simulink model "PLANTA_CODESYS"  (R2024b)
settings: Solver=FixedStepAuto  StartTime=0.0  StopTime=inf  FixedStep=0.001  MaxStep=0.0005  RelTol=1e-4
undefined symbols (not defined in the file): A_hm, A_tm, at_breakpoints, b_ha, B_hm, b_ta, B_tm, bcx, bcy, bhd, bhEb, bhm, bt, btd, btm, btw, bwu, C_hm, C_tm, D_hm, D_tm, DiscIntNeverNeededParam, dl_h_ini, dx_l_ini, dx_t_ini, dx_td_ini, dxt_max, dy_l_ini, g, Hc, ih, it, J_eqt, Jhd_hEb, Jhm_hb, Jtd, Jtm_tb, K_hsa, K_hsia, K_tsa, K_tsia, Kcy, Kd_table, ke_int, Ke_tita, ke_tita, ke_w, Ke_w, kp_pos, Kp_table, kp_w, kpos, Ktw, kwu, l_breakpoints, l_h_ini, Lh0, ml_breakpoints, Ms, Mt ... (+16)
libraries: simulink x11, spsEdgeDetectorLib x5, simulink_extras x2, opcualib x2, dspsigops x2, dspstat3 x1, vrlib x1, sldrtlib x1
(part 2 of 2)

== system PLANTA_CODESYS/PLANTA/Altura perfil obstaculos (A partir de posicion x_l) ==
  x_l : Inport
  Ajuste referencia : Constant  Value=30
  Calculo : MATLAB Function  TreatAsAtomicUnit=on
  Data Store Read : DataStoreRead  DataStoreName=y0_global  IndexOptions=Index vector (dialog)  Indices=1  OutputSizes=1
  Data Type Conversion : DataTypeConversion  OutDataTypeStr=int32  RndMeth=Ceiling  SaturateOnIntegerOverflow=off
  Gain1 : Gain  Gain=1/Wc
  Scope : Scope
  Scope1 : Scope
  Sum : Sum  Inputs=|++
  yc0_xl : Outport
  wires:
  Calculo/1(yc0_xt) -> Scope1/1, yc0_xl/1
  Data Store Read/1 -> Calculo/1(y0_array)
  Data Type Conversion/1 -> Scope/1, Calculo/2(index)
  Gain1/1 -> Data Type Conversion/1
  Ajuste referencia/1 -> Sum/2
  Sum/1 -> Gain1/1
  x_l/1 -> Sum/1

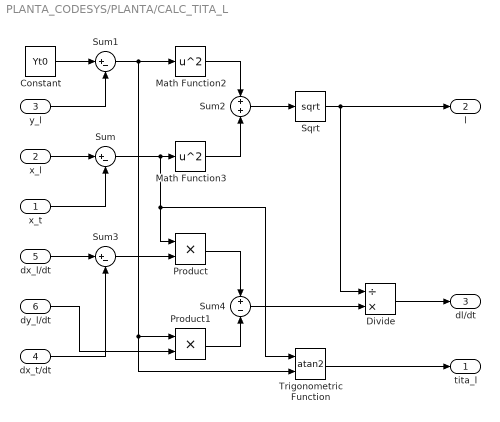
== system PLANTA_CODESYS/PLANTA/CALC_TITA_L ==
  x_t : Inport
  x_l : Inport  Port=2
  y_l : Inport  Port=3
  dx_t/dt : Inport  Port=4
  dx_l/dt : Inport  Port=5
  dy_l/dt : Inport  Port=6
  Constant : Constant  Value=Yt0
  Divide : Product  Inputs=/*
  Math Function2 : Math  Operator=square
  Math Function3 : Math  Operator=square
  Product : Product
  Product1 : Product
  Sqrt : Sqrt
  Sum : Sum  Inputs=|+-
  Sum1 : Sum  Inputs=|+-
  Sum2 : Sum  Inputs=+|+
  Sum3 : Sum  Inputs=|+-
  Sum4 : Sum  Inputs=+|-
  Trigonometric Function : Trigonometry  Operator=atan2
  tita_l : Outport
  l : Outport  Port=2
  dl/dt : Outport  Port=3
  wires:
  Product/1 -> Sum4/1
  Product1/1 -> Sum4/2
  x_l/1 -> Sum/1
  dx_t/dt/1 -> Sum3/2
  y_l/1 -> Sum1/2
  Sum/1 -> Product/1, Trigonometric Function/1, Math Function3/1
  Sqrt/1 -> l/1, Divide/1
  Sum2/1 -> Sqrt/1
  Sum4/1 -> Divide/2
  Sum1/1 -> Product1/1, Trigonometric Function/2, Math Function2/1
  Math Function2/1 -> Sum2/1
  dx_l/dt/1 -> Sum3/1
  x_t/1 -> Sum/2
  Constant/1 -> Sum1/1
  Sum3/1 -> Product/2
  dy_l/dt/1 -> Product1/2
  Math Function3/1 -> Sum2/2
  Trigonometric Function/1 -> tita_l/1
  Divide/1 -> dl/dt/1

== system PLANTA_CODESYS/PLANTA/FIN_CARRERA_IZAJE ==
  l_h : Inport
  Constant : Constant  Value=Yt0
  Constant1 : Constant  Value=-19.5
  Constant2 : Constant  Value=-20
  Constant3 : Constant  Value=49.5
  Constant4 : Constant  Value=50
  Relational Operator : RelationalOperator  Operator=<=  OutDataTypeStr=boolean  RndMeth=Simplest  InputSameDT=off
  Relational Operator1 : RelationalOperator  Operator=<=  OutDataTypeStr=boolean  RndMeth=Simplest  InputSameDT=off
  Relational Operator2 : RelationalOperator  OutDataTypeStr=boolean  RndMeth=Simplest  InputSameDT=off
  Relational Operator3 : RelationalOperator  OutDataTypeStr=boolean  RndMeth=Simplest  InputSameDT=off
  Sum : Sum  Inputs=|-+
  FC_INF : Outport
  FCE_INF : Outport  Port=2
  FC_SUP : Outport  Port=3
  FCE_SUP : Outport  Port=4
  wires:
  Sum/1 -> Relational Operator3/1, Relational Operator2/1, Relational Operator/1, Relational Operator1/1  "y_h"
  Relational Operator3/1 -> FCE_SUP/1
  Constant4/1 -> Relational Operator3/2
  Relational Operator2/1 -> FC_SUP/1
  Constant3/1 -> Relational Operator2/2
  Constant1/1 -> Relational Operator/2
  Constant2/1 -> Relational Operator1/2
  Relational Operator/1 -> FC_INF/1
  Constant/1 -> Sum/2
  Relational Operator1/1 -> FCE_INF/1
  l_h/1 -> Sum/1

== system PLANTA_CODESYS/PLANTA/Fin de carrera Carro ==
  x_t : Inport
  Constant : Constant  Value=-29.5
  Constant1 : Constant  Value=-30
  Constant2 : Constant  Value=49.5
  Constant3 : Constant  Value=50
  Relational Operator : RelationalOperator  Operator=<=  OutDataTypeStr=boolean  RndMeth=Simplest  InputSameDT=off
  Relational Operator1 : RelationalOperator  Operator=<=  OutDataTypeStr=boolean  RndMeth=Simplest  InputSameDT=off
  Relational Operator2 : RelationalOperator  OutDataTypeStr=boolean  RndMeth=Simplest  InputSameDT=off
  Relational Operator3 : RelationalOperator  OutDataTypeStr=boolean  RndMeth=Simplest  InputSameDT=off
  FC_IZQ : Outport
  FCE_IZQ : Outport  Port=2
  FC_DER : Outport  Port=3
  FCE_DER : Outport  Port=4
  wires:
  Relational Operator/1 -> FC_IZQ/1
  Constant1/1 -> Relational Operator1/2
  x_t/1 -> Relational Operator3/1, Relational Operator2/1, Relational Operator/1, Relational Operator1/1
  Relational Operator1/1 -> FCE_IZQ/1
  Constant2/1 -> Relational Operator2/2
  Relational Operator2/1 -> FC_DER/1
  Relational Operator3/1 -> FCE_DER/1
  Constant3/1 -> Relational Operator3/2
  Constant/1 -> Relational Operator/2

== system PLANTA_CODESYS/PLANTA/Fuerzas de tension de cable en Carro ==
  x_td : Inport
  dx_td : Inport  Port=2
  x_t : Inport  Port=3
  dx_t : Inport  Port=4
  Add : Sum  Inputs=+-
  Add1 : Sum  Inputs=+-
  Add2 : Sum
  Gain : Gain  Gain=Ktw
  Gain1 : Gain  Gain=btw
  F_tw : Outport
  wires:
  Add1/1 -> Gain1/1
  Add/1 -> Gain/1
  Gain1/1 -> Add2/2
  x_td/1 -> Add/1
  dx_t/1 -> Add1/2
  dx_td/1 -> Add1/1
  Gain/1 -> Add2/1
  Add2/1 -> F_tw/1
  x_t/1 -> Add/2

== system PLANTA_CODESYS/PLANTA/Masa de contenedor (A partir de posicion x_l) ==
  TLK : Inport
  x_l : Inport  Port=2
  masas_array : Inport  Port=3
  Ajuste referencia : Constant  Value=30
  Calculo : MATLAB Function  TreatAsAtomicUnit=on
  Data Type Conversion : DataTypeConversion  OutDataTypeStr=int32  RndMeth=Ceiling  SaturateOnIntegerOverflow=off
  Edge Detector : spsEdgeDetectorLib/Edge Detector  model=Falling  ic=0  Ts=-1
  Edge Detector1 : spsEdgeDetectorLib/Edge Detector  model=Rising  ic=0  Ts=-1
  Gain1 : Gain  Gain=1/Wc
  Product : Product
  S-R Flip-Flop : simulink_extras/Flip Flops/S-R Flip-Flop  initial_condition=0
  Sample and Hold : dspsigops/Sample and Hold  trig=Rising edge  initCond=0  latchinput=off
  Sum : Sum  Inputs=|++
  Unit Delay : UnitDelay  SampleTime=-1  HasFrameUpgradeWarning=on
  Mc_X : Outport
  wires:
  Data Type Conversion/1 -> Calculo/2(index)
  Gain1/1 -> Data Type Conversion/1
  Ajuste referencia/1 -> Sum/2
  Sum/1 -> Gain1/1
  x_l/1 -> Sum/1
  TLK/1 -> Unit Delay/1
  Edge Detector/1 -> S-R Flip-Flop/2
  Edge Detector1/1 -> S-R Flip-Flop/1
  S-R Flip-Flop/1 -> Sample and Hold/Trigger, Product/2
  Product/1 -> Mc_X/1
  Unit Delay/1 -> Edge Detector1/1, Edge Detector/1
  Calculo/1(Mc_X) -> Sample and Hold/1
  Sample and Hold/1 -> Product/1
  masas_array/1 -> Calculo/1(masas_array)

== system PLANTA_CODESYS/PLANTA/PERFIL_OBSTACULOS ==
  note: LIDAR
  x_t : Inport
  Ajuste distancia LIDAR : dspsigops/Variable Fractional Delay  mode=OBSOLETE  modeActive=Linear  L=4  FarrowL=4  R=10  alpha=1  dmax=100  InputProcessing=Columns as channels (frame based)  ic=0  noDFT=off  fallbackFIR=Clip to the minimum value necessary for centered kernel  fallbackFarrow=Clip to the minimum value necessary for centered kernel  roundingMode=Zero  overflowMode=off
  Ajuste referencia : Constant  Value=30
  Constant : Constant  Value=Yt0
  Data Type Conversion : DataTypeConversion  OutDataTypeStr=int32  RndMeth=Ceiling  SaturateOnIntegerOverflow=off
  Delay : Delay  DelayLength=1  InputProcessing=Columns as channels (frame based)  SampleTime=0.001
  Delay espacial : Constant  Value=3/Wc
  Gain : Gain  Gain=1/Wc
  Perfil obstaculos (ENTORNO) : FromWorkspace  VariableName=y0
  Posicion LIDAR : Constant  Value=3
  Sum : Sum  Inputs=|++
  Sum1 : Sum  Inputs=|++
  Sum2 : Sum  Inputs=+-|
  sensor : MATLAB Function  TreatAsAtomicUnit=on
  yc0_xt : Outport
  wires:
  Delay/1 -> Sum1/1
  Sum/1 -> Gain/1
  Constant/1 -> Sum2/1
  Sum2/1 -> yc0_xt/1
  Sum1/1 -> Sum/1
  Delay espacial/1 -> Ajuste distancia LIDAR/2
  Ajuste distancia LIDAR/1 -> Sum2/2
  Data Type Conversion/1 -> sensor/2(index)
  Perfil obstaculos (ENTORNO)/1 -> sensor/1(y0_array)
  sensor/1(distancia) -> Ajuste distancia LIDAR/1
  Posicion LIDAR/1 -> Sum1/2
  Gain/1 -> Data Type Conversion/1
  x_t/1 -> Delay/1
  Ajuste referencia/1 -> Sum/2

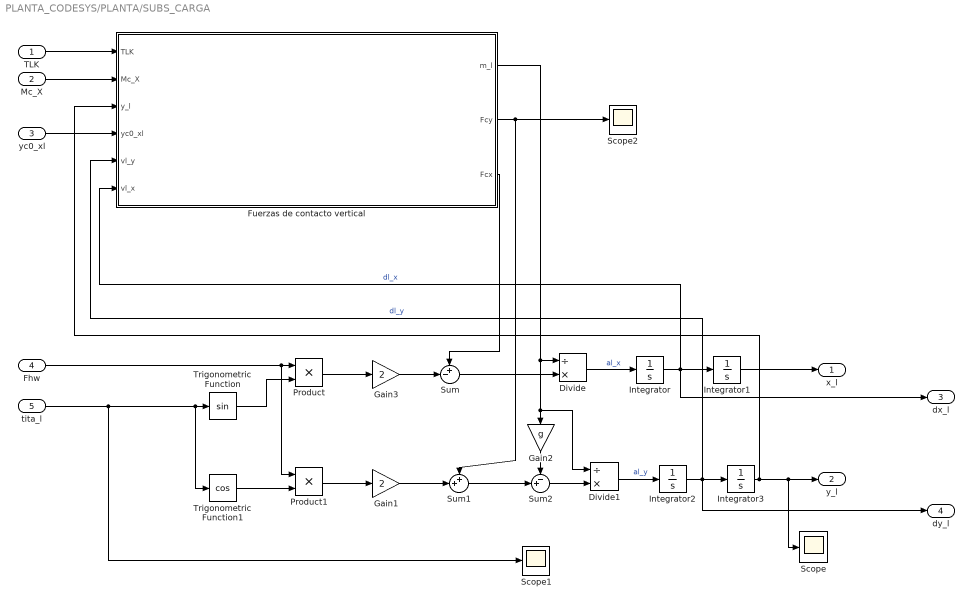
== system PLANTA_CODESYS/PLANTA/SUBS_CARGA ==
  TLK : Inport
  Mc_X : Inport  Port=2
  yc0_xl : Inport  Port=3
  Fhw : Inport  Port=4
  tita_l : Inport  Port=5
  Divide : Product  Inputs=/*
  Divide1 : Product  Inputs=/*
  Fuerzas de contacto vertical : Subsystem
  Gain1 : Gain  Gain=2
  Gain2 : Gain  Gain=g
  Gain3 : Gain  Gain=2
  Integrator : Integrator  InitialCondition=dx_l_ini
  Integrator1 : Integrator  InitialCondition=x_l_ini
  Integrator2 : Integrator  InitialCondition=dy_l_ini
  Integrator3 : Integrator  InitialCondition=y_l_ini
  Product : Product
  Product1 : Product
  Scope : Scope
  Scope1 : Scope
  Scope2 : Scope
  Sum : Sum  Inputs=+-|
  Sum1 : Sum  Inputs=++|
  Sum2 : Sum  Inputs=-+|
  Trigonometric Function : Trigonometry
  Trigonometric Function1 : Trigonometry  Operator=cos
  x_l : Outport
  y_l : Outport  Port=2
  dx_l : Outport  Port=3
  dy_l : Outport  Port=4
  wires:
  Divide1/1 -> Integrator2/1  "al_y"
  Sum2/1 -> Divide1/2
  Integrator2/1 -> dy_l/1, Integrator3/1, Fuerzas de contacto vertical/5(vl_y)  "dl_y"
  Fhw/1 -> Product1/1, Product/1
  Integrator3/1 -> Scope/1, y_l/1, Fuerzas de contacto vertical/3(y_l)
  Divide/1 -> Integrator/1  "al_x"
  Product1/1 -> Gain1/1
  Sum/1 -> Divide/2
  Fuerzas de contacto vertical/1(m_l) -> Divide/1, Divide1/1, Gain2/1
  Gain1/1 -> Sum1/2
  Trigonometric Function1/1 -> Product1/2
  Fuerzas de contacto vertical/3(Fcx) -> Sum/1
  Gain2/1 -> Sum2/1
  Integrator/1 -> dx_l/1, Fuerzas de contacto vertical/6(vl_x), Integrator1/1  "dl_x"
  Fuerzas de contacto vertical/2(Fcy) -> Sum1/1, Scope2/1
  tita_l/1 -> Scope1/1, Trigonometric Function1/1, Trigonometric Function/1
  Product/1 -> Gain3/1
  yc0_xl/1 -> Fuerzas de contacto vertical/4(yc0_xl)
  Trigonometric Function/1 -> Product/2
  Integrator1/1 -> x_l/1
  Sum1/1 -> Sum2/2
  Gain3/1 -> Sum/2
  Mc_X/1 -> Fuerzas de contacto vertical/2(Mc_X)
  TLK/1 -> Fuerzas de contacto vertical/1(TLK)

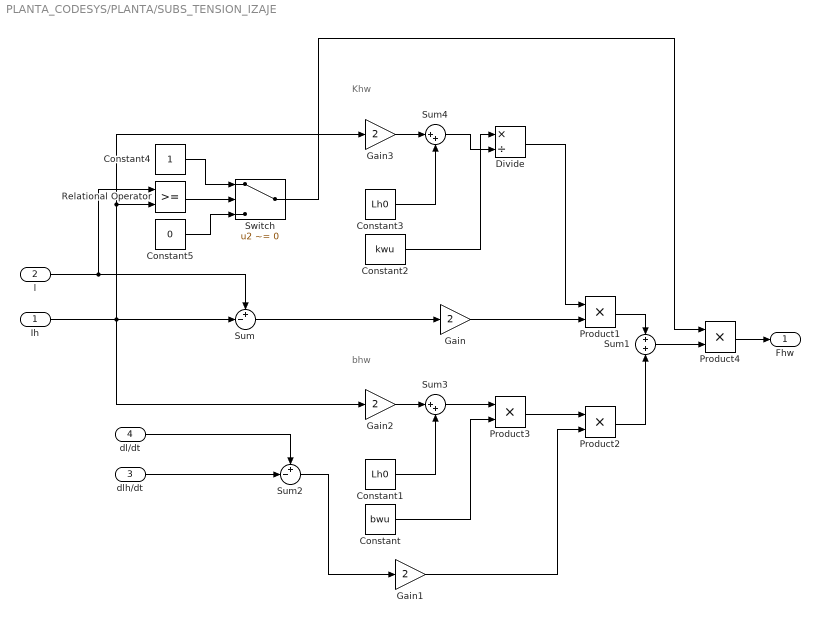
== system PLANTA_CODESYS/PLANTA/SUBS_TENSION_IZAJE ==
  note: Khw
  note: bhw
  Ih : Inport
  l : Inport  Port=2
  dlh/dt : Inport  Port=3
  dl/dt : Inport  Port=4
  Constant : Constant  Value=bwu
  Constant1 : Constant  Value=Lh0
  Constant2 : Constant  Value=kwu
  Constant3 : Constant  Value=Lh0
  Constant4 : Constant  OutDataTypeStr=double
  Constant5 : Constant  Value=0  OutDataTypeStr=double
  Divide : Product  Inputs=*/
  Gain : Gain  Gain=2
  Gain1 : Gain  Gain=2
  Gain2 : Gain  Gain=2  OutDataTypeStr=Inherit: Inherit via back propagation
  Gain3 : Gain  Gain=2  OutDataTypeStr=Inherit: Inherit via back propagation
  Product{1..4} (4 alike) : Product
  Relational Operator : RelationalOperator  OutDataTypeStr=boolean  RndMeth=Simplest  InputSameDT=off
  Sum : Sum  Inputs=+-|
  Sum1 : Sum  Inputs=+|+
  Sum2 : Sum  Inputs=+-|
  Sum3 : Sum  Inputs=|++
  Sum4 : Sum  Inputs=|++
  Switch : Switch  Criteria=u2 ~= 0  SaturateOnIntegerOverflow=off  InputSameDT=off
  Fhw : Outport
  wires:
  l/1 -> Sum/1, Relational Operator/1
  Constant4/1 -> Switch/1
  dlh/dt/1 -> Sum2/2
  Sum/1 -> Gain/1
  Product2/1 -> Sum1/2
  Sum1/1 -> Product4/2
  Gain/1 -> Product1/2
  Product3/1 -> Product2/1
  Sum4/1 -> Divide/2
  Sum2/1 -> Gain1/1
  Divide/1 -> Product1/1
  Product1/1 -> Sum1/1
  dl/dt/1 -> Sum2/1
  Constant/1 -> Product3/2
  Sum3/1 -> Product3/1
  Gain3/1 -> Sum4/1
  Ih/1 -> Gain2/1, Sum/2, Relational Operator/2, Gain3/1
  Constant1/1 -> Sum3/2
  Constant3/1 -> Sum4/2
  Relational Operator/1 -> Switch/2
  Switch/1 -> Product4/1
  Constant2/1 -> Divide/1
  Gain1/1 -> Product2/2
  Gain2/1 -> Sum3/1
  Constant5/1 -> Switch/3
  Product4/1 -> Fhw/1

== system PLANTA_CODESYS/PLANTA/Traslacion del carro ==
  F_tw : Inport
  F_hw : Inport  Port=2
  theta_l : Inport  Port=3
  Gain : Gain  Gain=2
  Gain1 : Gain  Gain=bt
  Gain2 : Gain  Gain=1/Mt
  Integrator : Integrator  InitialCondition=dx_t_ini
  Integrator1 : Integrator  InitialCondition=x_t_ini
  Product : Product
  Sin : Trigonometry
  Sum : Sum  Inputs=++-
  x_t : Outport
  dx_t : Outport  Port=2
  wires:
  Gain1/1 -> Sum/3
  Integrator1/1 -> x_t/1
  theta_l/1 -> Sin/1
  Sin/1 -> Product/2
  Sum/1 -> Gain2/1
  F_tw/1 -> Sum/1
  F_hw/1 -> Product/1
  Gain/1 -> Sum/2
  Integrator/1 -> dx_t/1, Gain1/1, Integrator1/1
  Product/1 -> Gain/1
  Gain2/1 -> Integrator/1  "ddx_t"

== system PLANTA_CODESYS/Nivel 2 - Control Regulatorio + Obs1/Observador_Control_Posicion/Fuerzas de tension de cable en Carro ==
  x_td : Inport
  dx_td : Inport  Port=2
  x_t : Inport  Port=3
  dx_t : Inport  Port=4
  Add : Sum  Inputs=+-
  Add1 : Sum  Inputs=+-
  Add2 : Sum
  Gain : Gain  Gain=Ktw
  Gain1 : Gain  Gain=btw
  F_tw : Outport
  wires:
  Add1/1 -> Gain1/1
  Add/1 -> Gain/1
  Gain1/1 -> Add2/2
  x_td/1 -> Add/1
  dx_t/1 -> Add1/2
  dx_td/1 -> Add1/1
  Gain/1 -> Add2/1
  Add2/1 -> F_tw/1
  x_t/1 -> Add/2

== system PLANTA_CODESYS/Nivel 2 - Control Regulatorio + Obs1/Observador_Control_Posicion/Observador ==
  x_td : Inport
  T_tm* : Inport  Port=2
  Discrete-Time Integrator : DiscreteIntegrator  InitialCondition=x_td_ini  SampleTime=T_s2  ICPrevOutput=DiscIntNeverNeededParam  ICPrevScaledInput=DiscIntNeverNeededParam
  Discrete-Time Integrator1 : DiscreteIntegrator  InitialCondition=dx_td_ini  SampleTime=T_s2  ICPrevOutput=DiscIntNeverNeededParam  ICPrevScaledInput=DiscIntNeverNeededParam
  Gain : Gain  Gain=rtd/J_eqt
  Gain1 : Gain  Gain=Ke_tita
  Gain2 : Gain  Gain=Ke_w
  Gain3 : Gain  Gain=it
  Sum1 : Sum  Inputs=|++
  Sum2 : Sum  Inputs=|++
  Sum3 : Sum  Inputs=+-|
  dx_td_obs : Outport
  wires:
  T_tm*/1 -> Gain3/1
  Gain/1 -> Sum1/1
  Sum1/1 -> Discrete-Time Integrator1/1  "ddx_td_obs"
  x_td/1 -> Sum3/1
  Sum3/1 -> Gain2/1, Gain1/1
  Gain1/1 -> Sum2/2
  Gain2/1 -> Sum1/2
  Sum2/1 -> Discrete-Time Integrator/1, dx_td_obs/1
  Gain3/1 -> Gain/1
  Discrete-Time Integrator/1 -> Sum3/2
  Discrete-Time Integrator1/1 -> Sum2/1

== system PLANTA_CODESYS/Nivel 2 - Control Regulatorio + Obs1/Observador_Control_Posicion/Subsystem ==
  xt_obs : Inport
  xt_ref : Inport  Port=2
  Discrete Derivative : simulink/Discrete/Discrete Derivative  Commented=on  gainval=1.0  ICPrevScaledInput=0.0  OutMin=[]  OutMax=[]  OutDataType=fixdt(1, 16)  OutScaling=2^-10  DoSatur=off
  Gain : Gain  Gain=kp_pos
  Gain1 : Gain  Commented=on  Gain=kp_w
  Sum : Sum  Inputs=|++
  Sum1 : Sum  Inputs=|-+
  dxt_pos : Outport
  wires:
  xt_ref/1 -> Sum1/2
  Sum1/1 -> Discrete Derivative/1, Gain/1  "e_pos"
  Gain1/1 -> Sum/2  "dxt_pos"
  Sum/1 -> dxt_pos/1
  xt_obs/1 -> Sum1/1
  Discrete Derivative/1 -> Gain1/1
  Gain/1 -> Sum/1  "dxt_pos"

== system PLANTA_CODESYS/Nivel 2 - Control Regulatorio + Obs1/Observador_Control_Posicion/Traslacion del carro ==
  F_tw : Inport
  F_hw : Inport  Port=2
  theta_l : Inport  Port=3
  Discrete-Time Integrator : DiscreteIntegrator  InitialCondition=dx_t_ini  SampleTime=T_s2  ICPrevOutput=DiscIntNeverNeededParam  ICPrevScaledInput=DiscIntNeverNeededParam
  Discrete-Time Integrator1 : DiscreteIntegrator  InitialCondition=x_t_ini  SampleTime=T_s2  ICPrevOutput=DiscIntNeverNeededParam  ICPrevScaledInput=DiscIntNeverNeededParam
  Gain : Gain  Gain=2
  Gain1 : Gain  Gain=bt
  Gain2 : Gain  Gain=1/Mt
  Product : Product
  Sin : Trigonometry
  Sum : Sum  Inputs=++-
  x_t : Outport
  dx_t : Outport  Port=2
  wires:
  Gain1/1 -> Sum/3
  theta_l/1 -> Sin/1
  Sin/1 -> Product/2
  Sum/1 -> Gain2/1
  F_tw/1 -> Sum/1
  F_hw/1 -> Product/1
  Gain/1 -> Sum/2
  Product/1 -> Gain/1
  Gain2/1 -> Discrete-Time Integrator/1  "ddx_t"
  Discrete-Time Integrator/1 -> Discrete-Time Integrator1/1, Gain1/1, dx_t/1
  Discrete-Time Integrator1/1 -> x_t/1

== system PLANTA_CODESYS/PLANTA/Accionamiento de Izaje/Freno ==
  w_hm : Inport
  BRK_h : Inport  Port=2
  Constant : Constant  Value=0
  Gain5 : Gain  Gain=-bhd
  Saturation : Saturate  UpperLimit=Thb_Max  LowerLimit=-Thb_Max
  Scope : Scope
  Switch : Switch  Criteria=u2 > Threshold  SaturateOnIntegerOverflow=off  InputSameDT=off
  T_hb : Outport
  wires:
  Gain5/1 -> Saturation/1
  BRK_h/1 -> Switch/2
  Saturation/1 -> Switch/3
  Constant/1 -> Switch/1
  w_hm/1 -> Gain5/1
  Switch/1 -> Scope/1, T_hb/1

== system PLANTA_CODESYS/PLANTA/Accionamiento de Izaje/Freno Emergencia ==
  w_hd : Inport
  BRK_hE : Inport  Port=2
  Constant : Constant  Value=0
  Gain5 : Gain  Gain=-bhEb
  Saturation : Saturate  UpperLimit=ThEb_Max  LowerLimit=-ThEb_Max
  Switch : Switch  Criteria=u2 > Threshold  SaturateOnIntegerOverflow=off  InputSameDT=off
  T_hEB : Outport
  wires:
  Gain5/1 -> Saturation/1
  BRK_hE/1 -> Switch/2
  Saturation/1 -> Switch/3
  Constant/1 -> Switch/1
  w_hd/1 -> Gain5/1
  Switch/1 -> T_hEB/1

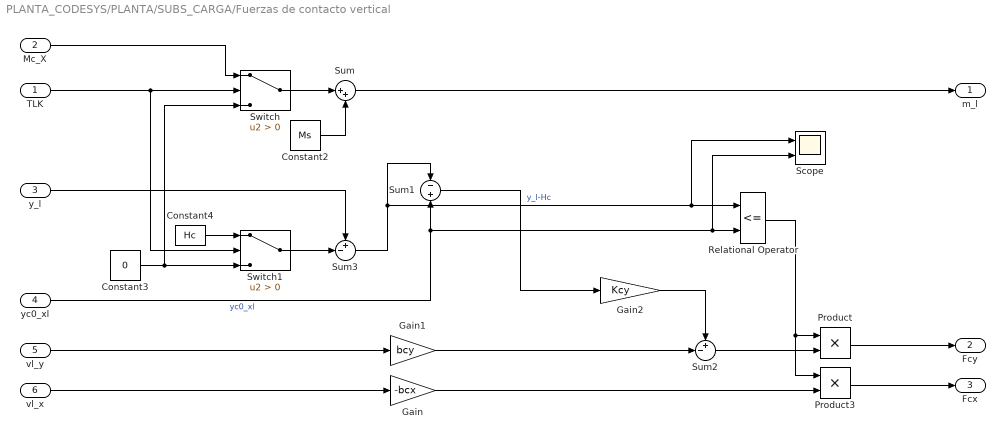
== system PLANTA_CODESYS/PLANTA/SUBS_CARGA/Fuerzas de contacto vertical ==
  TLK : Inport
  Mc_X : Inport  Port=2
  y_l : Inport  Port=3
  yc0_xl : Inport  Port=4
  vl_y : Inport  Port=5
  vl_x : Inport  Port=6
  Constant2 : Constant  Value=Ms
  Constant3 : Constant  Value=0
  Constant4 : Constant  Value=Hc
  Gain : Gain  Gain=-bcx
  Gain1 : Gain  Gain=bcy
  Gain2 : Gain  Gain=Kcy
  Product : Product
  Product3 : Product
  Relational Operator : RelationalOperator  Operator=<=  OutDataTypeStr=boolean  RndMeth=Simplest  InputSameDT=off
  Scope : Scope  NumInputPorts=2
  Sum : Sum  Inputs=|++
  Sum1 : Sum  Inputs=-|+
  Sum2 : Sum  Inputs=+-|
  Sum3 : Sum  Inputs=+-|
  Switch : Switch  Criteria=u2 > Threshold  SaturateOnIntegerOverflow=off  InputSameDT=off
  Switch1 : Switch  Criteria=u2 > Threshold  SaturateOnIntegerOverflow=off  InputSameDT=off
  m_l : Outport
  Fcy : Outport  Port=2
  Fcx : Outport  Port=3
  wires:
  TLK/1 -> Switch/2, Switch1/2
  Gain1/1 -> Sum2/2
  Switch/1 -> Sum/1
  Constant3/1 -> Switch1/3, Switch/3
  yc0_xl/1 -> Scope/2, Relational Operator/2, Sum1/2  "yc0_xl"
  Constant2/1 -> Sum/2
  Sum3/1 -> Scope/1, Relational Operator/1, Sum1/1  "y_l-Hc"
  Sum2/1 -> Product/2
  vl_y/1 -> Gain1/1
  Gain/1 -> Product3/2
  Switch1/1 -> Sum3/2
  Constant4/1 -> Switch1/1
  vl_x/1 -> Gain/1
  Gain2/1 -> Sum2/1
  Sum1/1 -> Gain2/1
  Sum/1 -> m_l/1
  y_l/1 -> Sum3/1
  Mc_X/1 -> Switch/1
  Product/1 -> Fcy/1
  Product3/1 -> Fcx/1
  Relational Operator/1 -> Product3/1, Product/1

== matlab function PLANTA_CODESYS/Actualizar perfil/Enabled Subsystem/Actualiza perfil ==
  data: index input; y0_actualizado output; y0 input; Hc input
function y0_actualizado = fcn(index,y0,Hc)
y0_anterior=y0;
if (abs(index)>0 && abs(index)<=32)
y0_anterior(abs(index))=y0_anterior(abs(index))+Hc*sign(index);
y0_actualizado=y0_anterior;
else
y0_actualizado=y0;
end

== matlab function PLANTA_CODESYS/Nivel 2 - Control Regulatorio + Obs/Controlador de balanceo/MATLAB Function ==
  data: xt0 input; Kp output; vt0 input; th0 input; w0 input; Ftw0 input; Mt0 input; ml0 input; l0 input; bt0 input; g0 input; Kd output
function [Kp, Kd] = jacob(xt0,vt0,th0,w0,Ftw0,Mt0,ml0,l0,bt0,g0)

syms xt vt th w Ftw real
syms Mt ml l bt g_sym real

%%Linealizacion Jacobiana 

% Estados y entrada
x = [xt; vt; th; w];
u = Ftw;

% Definiciones auxiliares
Dx  = Mt + ml*sin(th)^2;
Nx = Ftw - bt*vt + ml*l*w^2*sin(th) + ml*g_sym*sin(th)*cos(th);
Nth = -(Mt+ml*sin(th)^2)*g_sym*sin(th)-cos(th)*(Ftw-bt*vt+ml*l*w^2*sin(th)+ml*g_sym*sin(th)*cos(th));
Dth = l*(Mt+ml*sin(th)^2);

% Dinámica
f1 = vt;
f2 = Nx / Dx;
f3 = w;
f4 = Nth / Dth;

f = [f1; f2; f3; f4];

% Jacobianos
A = jacobian(f, x);
B = jacobian(f, u);

% (opcional) simplificación
A = simplify(A);
B = simplify(B);

% Modelo LPV evaluado en el punto de operacion
A0 = subs(A, {xt,vt,th,w,Ftw,Mt,ml,l,bt,g_sym}, {xt0,vt0,th0,w0,Ftw0,Mt0,ml0,l0,bt0,g0});
B0 = subs(B, {xt,vt,th,w,Ftw,Mt,ml,l,bt,g_sym}, {xt0,vt0,th0,w0,Ftw0,Mt0,ml0,l0,bt0,g0});

%% Buscamos la dinamica natural del sistema
% Autovalores de la matriz A0
lambda = eig(double(A0));

% Ordenar por real(lambda) (más cercano a 0 -> dominante)
[~, idx] = sort(real(lambda), 'descend'); % mayor real -> más lento (menos negativo)
lambda_ord = lambda(idx);

% Seleccionar el primer autovalor
lambda_dom = lambda_ord(1);

% Si es complejo (par), buscar su conjugado y calcular wn_la
if imag(lambda_dom) ~= 0
    sigma = real(lambda_dom);
    wd = abs(imag(lambda_dom));
    wn_la = sqrt(sigma^2 + wd^2);
    dseta = -sigma / wn_la;
else
    % polo real dominante
    sigma = real(lambda_dom);   % negativo para estable
    wn_la = abs(sigma);       % uso de |sigma| como medida de velocidad
    dseta = 1;              % no aplica exactamente, placeholder
end

%% Obtencion de Funcion de transferencia
syms Kp Kd s real

Gc = Kp+Kd*s;

% Selección de salida y vector que representa la acción de delta-theta
C = [0 1 0 0];            % salida y = delta v_t
a_theta = A0(:,3);        % influencia de delta theta como "entrada"

%Para encontrar la funcion de transferencia
SI_A0 = s*eye(4) - A0;
Gp = simplify( C * inv(SI_A0)* B(:,1));  % TF de la planta

% Separar numerador y denominador simbólicos (opcional)
% [numG, denG] = numden(Gp);
% numG = simplify(expand(numG));
% denG = simplify(expand(denG));

% 
% Gct = (1.7024e+04)/(s^2)+(2.2754e+04)/s+(1.0849e+04);
% Gct = simplify(Gct);
% 
% Gcb = Gp/(1+Gct*Gc*Gp); 

Gcb = Gp/(1+Gc*Gp)
Gcb = simplify(Gcb);
[~, denGcb] = numden(Gcb);
denGcb = expand(denGcb);

%% Diseño por amortiguamiento crítico
% Usamos una wn mayor a la de lazo abierto
wn = 1.5*wn_la;

% Polinomio dominante de segundo orden crítico
P_dom = s^2 + 2*wn*s + wn^2;

% Polos no dominantes (rápidos)
alpha = 5*wn;
beta = 6*wn;
P_des = expand(P_dom * (s + alpha) * (s + beta));

% Polinomio del lazo cerrado
P_lc = denGcb;

% % Igualación de coeficientes
% Pdiff = (expand(D_lc - D_des));
% coeffs_vec = coeffs(Pdiff, s);
% eqs = coeffs_vec == 0;

% Forma robusta: extraer polinomio en vector
% [~,D_des_p] = numden(D_des);
% poly_des = expand(D_des);

% Igualación por coeficientes (grado 4 -> 5 ecuaciones)
coeffs_lc = coeffs(P_lc,s,'All');
coeffs_des = coeffs(P_des, s, 'All');

% alinear longitudes rellenando con ceros si es necesario
nL = length(coeffs_lc); nD = length(coeffs_des);
n = max(nL, nD);
coeffs_lc = [zeros(1,n-nL), coeffs_lc];
coeffs_des = [zeros(1,n-nD), coeffs_des];

% formar sistema de ecuaciones (vectorial)
eqs = coeffs_lc - coeffs_des;
eqs = simplify(eqs);           % ecuaciones simbólicas

% Resolver simbólicamente Kp, Kd
sol = solve(eqs, [Kp Kd], 'Real', true);

% recoger soluciones posibles
Kp_sol = sol.Kp;
Kd_sol = sol.Kd;

% % Si solve devuelve múltiples soluciones, filtrar:
% found = false;
% Kp = NaN; Kd = NaN; wn = NaN;
%     for i = 1:length(wn_sym)
%         try
%             wn_i = double(wn_sym(i));
%             Kp_i = double(Kp_sym(i));
%             Kd_i = double(Kd_sym(i));
%         catch
%             continue;
%         end
%         if ~isreal(wn_i) || wn_i <= 0 || ~isreal(Kp_i) || ~isreal(Kd_i)
%             continue;
%         end
%         % comprobar estabilidad del lazo cerrado
%         poly_lc_sub = double(subs(poly_lc, {Kp,Kd,wn}, {Kp_i,Kd_i,wn_i}));
%         % opcional: comprobar raices todas en LHP
%         coeff_vec = sym2poly(poly_lc_sub);
%         if isempty(coeff_vec)
%             continue;
%         end
%         rts = roots(coeff_vec);
%         if all(real(rts) < 0)
%             Kp = Kp_i; Kd = Kd_i; wn = wn_i;
%             found = true;
%         end
%     end
% 
%     if ~found
%         warning('No se encontró solución válida para Kp,Kd,wn con los criterios dados.');
%     end

end

== matlab function PLANTA_CODESYS/Nivel 2: Control Regulatorio1 ==
  data: Fhw input; T_tm output; T_hm output; dx_tref input; m_l input; BC input; dlh_ref input; l_h input; dl_h input; theta input; ddx_t_ref input; x_td input; dx_td input; xt_ref input; l_breakpoints parameter; ml_breakpoints parameter; at_breakpoints parameter; Kp_table parameter; Kd_table parameter
function [T_tm, T_hm]  = Nivel2(Fhw,dx_tref,m_l,BC,dlh_ref,l_h,dl_h,theta,ddx_t_ref, x_td, dx_td,xt_ref,l_breakpoints, ml_breakpoints, at_breakpoints, Kp_table, Kd_table)

%% PARAMETROS

% Datos generales
g = 9.80665;            % Aceleración gravitatoria [m/s^2]

% Accionamiento del Sistema de Izaje
tauhm = 1.0e-3;               % Constante de tiempo del modulador de torque en el motor [s]
Thm_Max = 20.0e3;             % Torque máximo de motorización/frenado regenerativo del motor [N*m]

% Accionamiento de Traslación del Carro
tautm = 1.0e-3;              % Constante de tiempo del modulador de torque (motor del carro) [s]
Ttm_Max = 4.0e3;             % Torque máximo de motorización/frenado regenerativo del motor [N*m]

% CN2 - DATOS GENERALES
T_s2=0.001; %Tiempo muestreo control nivel 2

% CN2 - PARAMETROS CONTROLADOR CARRO
b_ta = 1.084860000000000e+04;
K_tsa = 2.275381024560000e+04;
K_tsia = 1.702393005727008e+04;

% CN2 - PARAMETROS CONTROLADOR DE IZAJE
b_ha = -2.219636363636364e+04;
K_hsa = -8.441961938415557e+04;
K_hsia = -1.957032340849276e+05;

% CN2 - PARAMETROS OBSERVADOR CON CONTROL
%Observador
Ke_w = 10849.27;
Ke_tita = 209.27;
it = 30;
bt = 90;
Jtm_tb = 7;
Jtd = 1200;
rtd = 0.5;
Mt = 30000;
Ktw = 480000;
btw = 3000;
%Controlador
n = 2.5;
kp_pos = 0.15;
kp_w = n * kp_pos;


%% PROGRAM - MAIN

%VAR
persistent dx_td_obs_ant dxt_cp_ant ddxt_ant T_tm_out_ant;

if isempty(dx_td_obs_ant)
    dx_td_obs_ant = 0;
    dxt_cp_ant = 0;
    ddxt_ant = 0;
    T_tm_out_ant=0;
end

%BEGIN
if (BC==1)
    dx_tref_balanceo=controlBalanceo(m_l,l_h,ddxt_ant,ddx_t_ref,theta);
else
    dx_tref_balanceo=0;
end

[ddxt,dxt_pos,dx_td_obs]=observadorControl(T_tm_out_ant, x_td, xt_ref, theta, Fhw);

%Calculo de T_tm
T_tm_consig=controlCarro(dx_td,dx_tref+dx_tref_balanceo,b_ta,K_tsa,K_tsia);
T_tm_out=moduladorTorqueCarro(T_tm_consig);

%Calculo de T_hm
T_hm_consig=controlIzaje(dl_h,dlh_ref,b_ha,K_hsa,K_hsia);
T_hm_out=moduladorTorqueIzaje(T_hm_consig);

dxt_cp_ant = dxt_pos;
ddxt_ant = ddxt;
dx_td_obs_ant = dx_td_obs;
T_tm_out_ant = T_tm_out;
%OUTPUT
T_tm=T_tm_out;
T_hm=T_hm_out;

%% FUNCTION BLOCK - CONTROLADOR CARRO
function T_tm_consig=controlCarro(dx_t,dx_tref,b_ta,K_tsa,K_tsia)
    persistent error_prop_prev error_int_prev
    if isempty(error_prop_prev)
            error_prop_prev = 0;
            error_int_prev = 0;
    end
        error_t = dx_tref - dx_t;
        error_p = error_prop_prev + error_t*T_s2;
        error_i = error_int_prev + error_p*T_s2;
        T_tm_consig = K_tsia*error_i + K_tsa*error_p + b_ta*error_t;
        error_prop_prev = error_p;
        error_int_prev = error_i;
end
%% FUNCTION BLOCK - OBSERVADOR
function dx_td_obs=observador(x_td_real, T_tm_consigna)
    persistent int1_prev int2_prev 
    if isempty(int1_prev)
            int1_prev = 0;
            int2_prev = 0;
    end

   
    error_obs_pos = x_td_real - int2_prev;
    torque_in = T_tm_consigna*it*rtd/(Jtd+Jtm_tb*it^2);
    ddx_td_obs = Ke_w*error_obs_pos + torque_in;
    int1_prev = int1_prev + ddx_td_obs*T_s2;
    dx_td_obs = int1_prev ;
    int2_prev = int2_prev + (dx_td_obs + error_obs_pos*Ke_tita)* T_s2;
    
end
%% FUNCTION BLOCK - FUERZAS DE TENSION DE CABLE EN CARRO
function F_tw=fuerzaTension(dx_td_obs, x_td_real, x_t_obs, dx_t_obs)
    F_tw = (x_td_real-x_t_obs)*Ktw+(dx_td_obs-dx_t_obs)*btw;
end

%% FUNCTION BLOCK - FUERZAS DE TENSION DE CABLE EN CARRO
function [x_t_obs,dx_t_obs]=traslacCarro(F_tw, F_hw, theta)
    persistent int1_prev int2_prev 
    if isempty(int1_prev)
            int1_prev = 0;
            int2_prev = 0;
    end
    if isempty(F_tw)
            F_tw = 0;
    end
    
    dx_t_obs = int1_prev;
    x_t_obs = int2_prev;

    ddxt_obs = (F_tw+F_hw*sin(theta)*2-bt*dx_t_obs)*(1/Mt);

    int1_prev = int1_prev+ddxt_obs*T_s2;

    int2_prev = int2_prev+dx_t_obs*T_s2;

end

%% FUNCTION BLOCK - CONTROL DE POSICION
    function dx_t_pos=controlPosicion(x_t_obs, x_t_ref)
        persistent error_pos_ant der1_ant
        error_pos = x_t_ref-x_t_obs;
        if isempty(error_pos_ant)
            error_pos_ant = error_pos;
            der1_ant = 0;
        end

        if isempty(x_t_obs)
            x_t_obs=0;
        end

        sum1 = kp_pos*error_pos;
        sum2 = kp_w*(error_pos-error_pos_ant)/T_s2;
        dx_t_pos = sum1+sum2;

        error_pos_ant = error_pos;
    end
%% FUNCTION BLOCK - OBSERVADOR CON CONTROL
    function [ddx_t,dx_t_pos,dx_td_obs]=observadorControl(T_tm_consigna, x_td_real, x_t_ref, theta, F_hw)
        % Fuerza del cable
        persistent xt_ant dxt_ant 

        if isempty(xt_ant)
            xt_ant = 0;
            dxt_ant = 0;
        end

        xt=xt_ant;
        dxt=dxt_ant;
        
        dx_td_obs = observador(x_td_real, T_tm_consigna);
        F_tw = fuerzaTension(dx_td_obs, x_td_real, xt, dxt);
        
        [xt, dxt] = traslacCarro(F_tw, F_hw, theta);
        ddx_t = (dxt-dxt_ant)/T_s2;
        dx_t_pos=controlPosicion(xt, x_t_ref);
        
        xt_ant = xt;
        dxt_ant = dxt;

    end
%% FUNCTION BLOCK - CONTROLADOR BALANCEO
function dx_tref_balanceo=controlBalanceo(ml,lh,at,a_t_ref,theta)
    persistent error_p_prev theta_ant
    if isempty(error_p_prev)
    error_p_prev = 0;
    theta_ant = 0;
    end
    %Calculamos theta_ref
    theta_ref=atan(-a_t_ref/g);
    %Saturamos los input para evitar extrapolacion
    ml_sat = min(max(ml, ml_breakpoints(1)), ml_breakpoints(end));
    lh_sat = min(max(lh, l_breakpoints(1)), l_breakpoints(end));
    at_sat = min(max(at, at_breakpoints(1)), at_breakpoints(end));
    
    %Calculamos Kp y Kd
    Kp = interpn(ml_breakpoints,l_breakpoints, at_breakpoints, ...
                 Kp_table, ml_sat, lh_sat,at_sat, 'linear');
    
    Kd = interpn(ml_breakpoints,l_breakpoints, at_breakpoints, ...
                 Kd_table,ml_sat, lh_sat,  at_sat, 'linear');

    %Controlador
    error_p= theta_ref - theta;
    error_d=(theta-theta_ant)/T_s2;
    dx_tref_balanceo=Kp*0.3*error_p+Kd*(0.3)*error_d;

    error_p_prev = error_p;
    theta_ant = theta;
end
%% FUNCTION BLOCK - CONTROLADOR IZAJE
function T_hm_consig=controlIzaje(dl_h,dl_href,b_ha,K_hsa,K_hsia)
    persistent error_prop_prev error_int_prev
    if isempty(error_prop_prev)
            error_prop_prev = 0;
            error_int_prev = 0;
    end
        error_t = dl_href - dl_h;
        error_p = error_prop_prev + error_t*T_s2;
        error_i = error_int_prev + error_p*T_s2;
        T_hm_consig = K_hsia*error_i + K_hsa*error_p + b_ha*error_t;
        error_prop_prev = error_p;
        error_int_prev = error_i;
end
%% FUNCTION BLOCK - MODULADOR DE TORQUE EQUIVALENTE CARRO
function T_tm=moduladorTorqueCarro(T_tm_consig)
    persistent T_tm_ant
    
    if isempty(T_tm_ant)
    T_tm_ant = 0;
    end
    
    T_tm_lim = min(Ttm_Max, max(-Ttm_Max, T_tm_consig));
    
    alpha = exp(-T_s2/tautm);
    
    T_tm = alpha*T_tm_ant + (1 - alpha)*T_tm_lim;
    
    T_tm_ant = T_tm;
end
%% FUNCTION BLOCK - MODULADOR DE TORQUE EQUIVALENTE IZAJE
function T_hm=moduladorTorqueIzaje(T_hm_consig)
    persistent T_hm_ant
    
    if isempty(T_hm_ant)
    T_hm_ant = 0;
    end
    
    T_hm_lim = min(Thm_Max, max(-Thm_Max, T_hm_consig));
    
    alpha = exp(-T_s2/tauhm);
    
    T_hm = alpha*T_hm_ant + (1 - alpha)*T_hm_lim;
    
    T_hm_ant = T_hm;
end
end

== matlab function PLANTA_CODESYS/PLANTA/PERFIL_OBSTACULOS/sensor ==
  data: y0_array input; distancia output; index input; Yt0 parameter
function distancia= mideDistancia(y0_array,index, Yt0)
distancia = Yt0-y0_array(index);

== matlab function PLANTA_CODESYS/PLANTA/Altura perfil obstaculos (A partir de posicion x_l)/Calculo ==
  data: y0_array input; yc0_xt output; index input
function yc0_xt= calcula_y0(y0_array,index)

if (index>0 && index<=32)
    yc0_xt =y0_array(index);
else
    yc0_xt=0;    
end

== matlab function PLANTA_CODESYS/LIDAR/sensor ==
  data: y0_array input; distancia output; index input; Yt0 parameter
function distancia= mideDistancia(y0_array,index, Yt0)


if (index>0 && index<=32)
    distancia = Yt0-y0_array(index);
else
   distancia = Yt0;
end

== stateflow chart PLANTA_CODESYS/Enclavamiento ==
  state Espera
  state Cambiar
    entry:
    output=(~output);
  (default) -> Espera
  Espera -> Cambiar : [input]
  Cambiar -> Espera : [input==0]
  data: input input; output output boolean =false

== stateflow chart PLANTA_CODESYS/Enclavamiento1 ==
  state Espera
  state Cambiar
    entry:
    output=(~output);
  (default) -> Espera
  Espera -> Cambiar : [input]
  Cambiar -> Espera : [input==0]
  data: input input; output output boolean =false

== matlab function PLANTA_CODESYS/Estimador de masa y velocidad/Velocidad max izaje ==
  data: M_l input; dxt_max output
function dxt_max = fcn(M_l)

Pnom=956.15e3; %Potencia nominal motor
g= 9.80665; %Acel gravitatoria

if (M_l>=65000)
    dxt_max = 1.5; %1.5 m/s
elseif (32500<=M_l)&&(M_l<65000)
    dxt_max = Pnom/(M_l*g);
elseif (M_l<32500)
    dxt_max=3; %3 m/s
else
    dxt_max = 1.5;

end

== matlab function PLANTA_CODESYS/PLANTA/Masa de contenedor (A partir de posicion x_l)/Calculo ==
  data: masas_array input; Mc_X output; index input
function Mc_X= calcula_Mc_X(masas_array,index)

if (index>0 && index<=32)
    Mc_X =masas_array(index);
else
    Mc_X=0;

end
